simulink model "D_20210914_Modell_Inbetriebnahme_BreakOutBox_Jetson"  (R2021a)
settings: Solver=ode1  StartTime=0.0  StopTime=500  FixedStep=Ts  RelTol=1e-3
PreLoadFcn:
  | pulsePeriod = 0.05;
  | 
  | Ts = 0.001;
  | 
  | FPGA_Frequency = 75000000;
  | 
  | ts_IO691 = 5e-3;
PostLoadFcn:
  | ewolfSetUp
InitFcn:
  | pulsePeriod = 0.05;
  | 
  | Ts = 0.001;
  | 
  | FPGA_Frequency = 75000000;
  | 
  | ts_IO691 = 5e-3;
StopFcn:
  | Simulink.sdi.clearPreferences;
  | if isfile(['sdi_view_',bdroot,'.mldatx'])
  | Simulink.sdi.view;
  | pause(3);
  | Simulink.sdi.loadView(['sdi_view_',bdroot,]);
  | end
values from neighbouring files (symbols this model uses):
  max_ac = 2    [ewolfSetUp.m]
  max_steer = 0.26    [ewolfSetUp.m]
  min_ac = -3    [ewolfSetUp.m]
  min_steer = -0.26    [ewolfSetUp.m]
  PredictionHorizon = 30    [ewolfSetUp.m]
undefined symbols (not defined in the file or in its folder): canChannel, DiscIntNeverNeededParam, Ended, HS, IO291, IO397, Single
libraries: lllalib x255, canmsglib x143, simulink x33, speedgoatlib_IO191 x5, speedgoatlib_IO291 x5, speedgoatlib_IO691 x3, slrealtimeiplib x2, simulink_extras x1, speedgoatlib_fpga_dio x1, speedgoatlib_fpga_quadrature x1, speedgoatlib_fpga x1, canlib x1
(part 1 of 7)
settings Model: SimulationMode=external  ExtModeEnableFloating=off  Creator=daniel.carretero  LastModifiedBy=gao
settings SolverCC: ConcurrentTasks=on  PositivePriorityOrder=on  AutoInsertRateTranBlk=on
settings DataIOCC: ReturnWorkspaceOutputs=off
settings OptimizationCC: BlockReduction=off  OptimizeBlockIOStorage=off
settings DebuggingCC: TasksWithSamePriorityMsg=none  UnconnectedInputMsg=none  UnconnectedOutputMsg=none  UnconnectedLineMsg=none
settings HardwareCC: ProdBitPerLong=64  ProdLongLongMode=on  ProdHWDeviceType=Intel->x86-64 (Linux 64)
settings RTWCC: Description=Simulink Real-Time  SystemTargetFile=slrealtime.tlc  TemplateMakefile=slrealtime_default_tmf  RTWVerbose=off  Toolchain=Simulink Real-Time Toolchain  BuildConfiguration=Faster Runs  CodeExecutionProfiling=on  TargetLang=C++

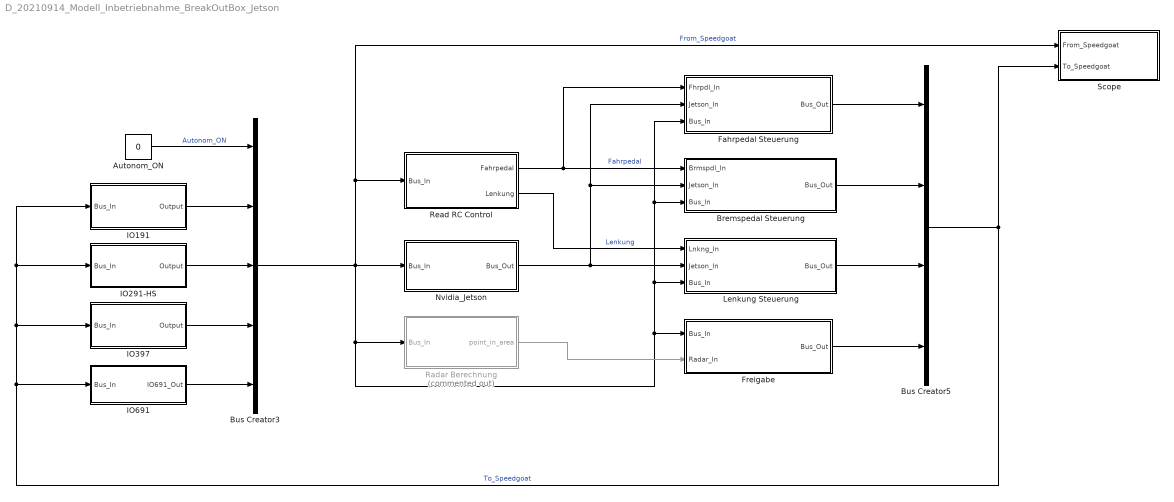
== system D_20210914_Modell_Inbetriebnahme_BreakOutBox_Jetson ==
  Autonom_ON : Constant  Value=0
  Bremspedal Steuerung : Subsystem
  Bus Creator3 : BusCreator  Inputs=5
  Bus Creator5 : BusCreator  Inputs=4
  Fahrpedal Steuerung : Subsystem
  Freigabe : Subsystem
  IO191 : Subsystem
  IO291-HS : Subsystem
  IO397 : Subsystem
  IO691 : Subsystem
  Lenkung Steuerung : Subsystem
  Nvidia_Jetson : Subsystem
  Radar Berechnung : Subsystem  Description=|  Commented=on
      | Extract radar data from CAN messages and create vector object with: 1788 fields:
      | 
      | 1. Timestamp
      | 2. cycle_count
      | 3. number of Objects
      | 4. radar timestamp_header
      | 5. CAN ID
      | +++++++++++++++++++++
      | % last point
      | 6. range
      | 7. az
      | 8. vr
      | 9. rcs
      | 10. el
      | ----------------------------------
      | % last point -1
      | 11. range
      | 12. az
      | 13. vr
      | 14. rcs
      | 15. el
      |  ...
      | 
      | empty points, all values == 0
  Read RC Control : Subsystem
  Scope : Subsystem
  wires:
  IO191/1(Output) -> Bus Creator3/2
  IO291-HS/1(Output) -> Bus Creator3/3
  IO397/1(Output) -> Bus Creator3/4
  Read RC Control/2(Lenkung) -> Lenkung Steuerung/1(Lnkng_In)  "Lenkung"
  Bus Creator3/1 -> Scope/1(From_Speedgoat), Read RC Control/1(Bus_In), Radar Berechnung/1(Bus_In), Fahrpedal Steuerung/3(Bus_In), Bremspedal Steuerung/3(Bus_In), Lenkung Steuerung/3(Bus_In), Freigabe/1(Bus_In), Nvidia_Jetson/1(Bus_In)  "From_Speedgoat"
  Read RC Control/1(Fahrpedal) -> Bremspedal Steuerung/1(Brmspdl_In), Fahrpedal Steuerung/1(Fhrpdl_In)  "Fahrpedal"
  IO691/1(IO691_Out) -> Bus Creator3/5
  Fahrpedal Steuerung/1(Bus_Out) -> Bus Creator5/1
  Lenkung Steuerung/1(Bus_Out) -> Bus Creator5/3
  Freigabe/1(Bus_Out) -> Bus Creator5/4
  Bremspedal Steuerung/1(Bus_Out) -> Bus Creator5/2
  Bus Creator5/1 -> IO191/1(Bus_In), IO291-HS/1(Bus_In), IO397/1(Bus_In), IO691/1(Bus_In), Scope/2(To_Speedgoat)  "To_Speedgoat"
  Nvidia_Jetson/1(Bus_Out) -> Fahrpedal Steuerung/2(Jetson_In), Bremspedal Steuerung/2(Jetson_In), Lenkung Steuerung/2(Jetson_In)
  Autonom_ON/1 -> Bus Creator3/1  "Autonom_ON"
  Radar Berechnung/1(point_in_area) -> Freigabe/2(Radar_In)

== system D_20210914_Modell_Inbetriebnahme_BreakOutBox_Jetson/Bremspedal Steuerung ==
  Brmspdl_In : Inport
  Jetson_In : Inport  Port=2
  Bus_In : Inport  Port=3
  1-D Lookup Table2 : Lookup_n-D  NumberOfTableDimensions=1  BreakpointsForDimension1=[min_ac max_ac]  Table=[-1 1]  InternalRulePriority=Speed  RndMeth=Simplest  InputSameDT=on
  AND3 : Logic  Inputs=3  AllPortsSameDT=off  OutDataTypeStr=boolean
  AND4 : Logic  Inputs=3  AllPortsSameDT=off  OutDataTypeStr=boolean
  Bus Creator : BusCreator  Inputs=2
  Bus Selector : BusSelector  OutputSignals=IO291_Out.IO291_Iso_DI.IO291_DI_CH1_NotAus_1,IO291_Out.IO291_Iso_DI.IO291_DI_CH2_NotAus_2,IO397_Out.IO397_DIO.IO397_DI_Ch8_Bremsaktuator_Hall_1,IO397_Out.IO397_DIO.IO397_DI_Ch9_Bremsaktuator_Hall_2,IO397_Out.IO397_QAD.IO397_QAD_Turns,Autonom_ON
  Bus Selector1 : BusSelector  OutputSignals=acceleration
  Gain : Gain  Gain=-1
  Moving Average : Subsystem
  Moving Average1 : Subsystem
  QAD Steuerung : Subsystem  Commented=on
  QAD Steuerung1 : Subsystem
  Saturation3 : Saturate  UpperLimit=0  LowerLimit=-1
  Switch : Switch  Criteria=u2 > Threshold  Threshold=0.5
  Bus_Out : Outport
  wires:
  Brmspdl_In/1 -> Switch/3
  Saturation3/1 -> Gain/1
  Bus_In/1 -> Bus Selector/1
  Bus Selector/2 -> AND4/2, AND3/2  "<IO291_DI_CH2_NotAus_2>"
  Bus Selector/1 -> AND4/1, AND3/1  "<IO291_DI_CH1_NotAus_1>"
  AND3/1 -> Bus Creator/1  "Bremsaktuator_1"
  AND4/1 -> Bus Creator/2  "Bremsaktuator_2"
  Bus Selector/5 -> QAD Steuerung/1(<QAD_Turns>)  "<IO397_QAD_Turns>"
  Gain/1 -> QAD Steuerung1/3(Brk), QAD Steuerung/2(u)
  Bus Selector/3 -> Moving Average/1(In)  "<IO397_DI_Ch8_Bremsaktuator_Hall_1>"
  Bus Selector/4 -> Moving Average1/1(In)  "<IO397_DI_Ch9_Bremsaktuator_Hall_2>"
  Moving Average/1(Hall_A) -> QAD Steuerung1/1(Hall_A)  "Hall_A"
  Moving Average1/1(Hall_B) -> QAD Steuerung1/2(Hall_B)  "Hall_B"
  QAD Steuerung1/1(Rel_1) -> AND3/3  "Rel_1"
  QAD Steuerung1/2(Rel_2) -> AND4/3  "Rel_2"
  Bus Creator/1 -> Bus_Out/1  "Brmskttr"
  Jetson_In/1 -> Bus Selector1/1
  Bus Selector1/1 -> 1-D Lookup Table2/1  "<acceleration>"
  Bus Selector/6 -> Switch/2  "<Autonom_ON>"
  Switch/1 -> Saturation3/1
  1-D Lookup Table2/1 -> Switch/1

== system D_20210914_Modell_Inbetriebnahme_BreakOutBox_Jetson/Fahrpedal Steuerung ==
  Fhrpdl_In : Inport
  Jetson_In : Inport  Port=2
  Bus_In : Inport  Port=3
  1-D Lookup Table : Lookup_n-D  NumberOfTableDimensions=1  BreakpointsForDimension1=[0:1]  Table=[0.8 5]  InternalRulePriority=Speed  RndMeth=Simplest  InputSameDT=on
  1-D Lookup Table1 : Lookup_n-D  NumberOfTableDimensions=1  BreakpointsForDimension1=[0:1]  Table=[0.4 2.5]  InternalRulePriority=Speed  RndMeth=Simplest  InputSameDT=on
  1-D Lookup Table2 : Lookup_n-D  NumberOfTableDimensions=1  BreakpointsForDimension1=[min_ac max_ac]  Table=[-1 1]  InternalRulePriority=Speed  RndMeth=Simplest  InputSameDT=on
  Bias1 : Bias
  Bias2 : Bias
  Bus Creator : BusCreator  Inputs=2
  Bus Selector : BusSelector  OutputSignals=acceleration
  Bus Selector1 : BusSelector  OutputSignals=Autonom_ON
  IC2 : InitialCondition  Value=0.8
  IC3 : InitialCondition  Value=0.4
  Saturation3 : Saturate  UpperLimit=1  LowerLimit=0
  Switch : Switch  Criteria=u2 > Threshold  Threshold=0.5
  Bus_Out : Outport
  wires:
  Bias1/1 -> Bus Creator/1  "Ausgabe_Gaspedal_FP_1_G"
  Bias2/1 -> Bus Creator/2  "Ausgabe_Gaspedal_FP_2_G"
  IC2/1 -> Bias1/1
  IC3/1 -> Bias2/1
  1-D Lookup Table/1 -> IC2/1
  Saturation3/1 -> 1-D Lookup Table1/1, 1-D Lookup Table/1
  1-D Lookup Table1/1 -> IC3/1
  Bus Creator/1 -> Bus_Out/1  "Fhrpdl"
  Jetson_In/1 -> Bus Selector/1
  Bus Selector/1 -> 1-D Lookup Table2/1  "<acceleration>"
  Bus_In/1 -> Bus Selector1/1
  Bus Selector1/1 -> Switch/2  "<Autonom_ON>"
  Fhrpdl_In/1 -> Switch/3
  Switch/1 -> Saturation3/1
  1-D Lookup Table2/1 -> Switch/1

== system D_20210914_Modell_Inbetriebnahme_BreakOutBox_Jetson/Freigabe ==
  Bus_In : Inport
  Radar_In : Inport  Port=2
  Bus Creator : BusCreator  Inputs=8
  Constant13 : Constant
  Constant8 : Constant  Value=0
  Freigabe : Subsystem
  Gain{4..9} (6 alike) : Gain
  Terminator : Terminator
  Totmann : Subsystem
  Bus_Out : Outport
  wires:
  Totmann/1(Totmann_Freigabe) -> Freigabe/2(Totmann_In)
  Bus_In/1 -> Freigabe/1(Bus_In), Totmann/1(Bus_In)
  Totmann/2(Totmann_LED) -> Gain4/1
  Gain4/1 -> Bus Creator/7  "LED_Totmann"
  Gain8/1 -> Bus Creator/3  "LG_FET_1_On"
  Gain9/1 -> Bus Creator/4  "LG_FET_2_On"
  Gain7/1 -> Bus Creator/2  "FP_FET_2_On"
  Gain5/1 -> Bus Creator/6  "Taster_Freigabe"
  Freigabe/1(Freigabe_Out) -> Gain5/1, Gain9/1, Gain8/1, Gain7/1, Gain6/1
  Constant8/1 -> Bus Creator/5  "Br_Licht_On"
  Gain6/1 -> Bus Creator/1  "FP_FET_1_On"
  Bus Creator/1 -> Bus_Out/1  "Freigabe"
  Constant13/1 -> Bus Creator/8  "USS_Reverse"
  Radar_In/1 -> Terminator/1

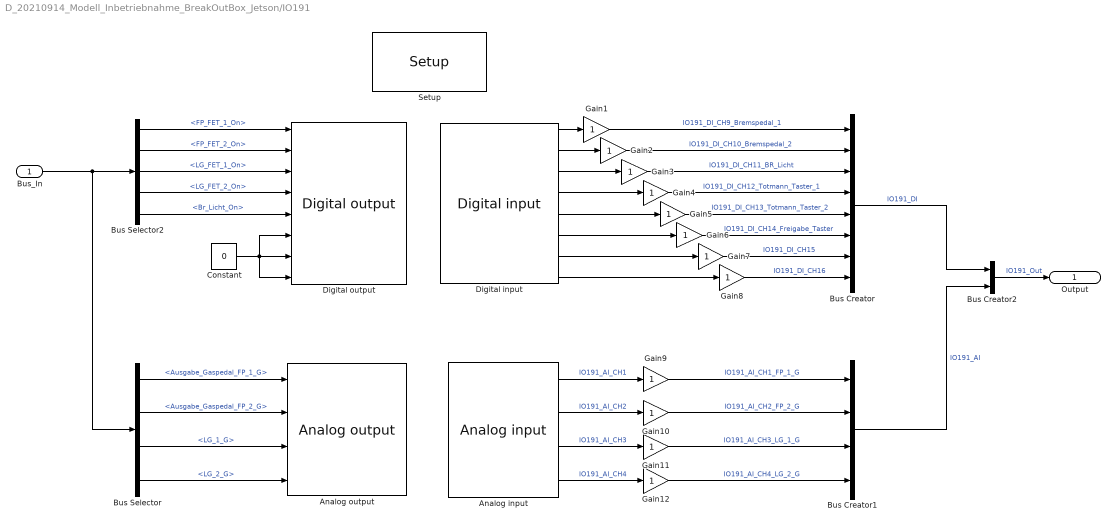
== system D_20210914_Modell_Inbetriebnahme_BreakOutBox_Jetson/IO191 ==
  Bus_In : Inport
  "Analog input " : speedgoatlib_IO191/Analog input   parModuleId=1  parSampleTime=Ts  parPciSlot=-1  parAdcChannels=[1 2 3 4]  parAdcMode=2  parAdcRanges=[4 4 4 4]  parAdcRate=100000  parAdcInitValues=[0 0]  parAdcResets=[1 1]
      settings: SourceProductName=Simulink Real-Time: Speedgoat I/O Blockset
  "Analog output " : speedgoatlib_IO191/Analog output   parModuleId=1  parSampleTime=Ts  parPciSlot=-1  parDacChannels=[1 2 3 4]  parModuleType=1  parDacRanges=[1 1 1 1]  parDacInitValues=[0 0 2.5 2.5]  parDacResets=[1 1 1 1]
      settings: SourceProductName=Simulink Real-Time: Speedgoat I/O Blockset
  Bus Creator : BusCreator  Inputs=8
  Bus Creator1 : BusCreator  Inputs=4
  Bus Creator2 : BusCreator  Inputs=2
  Bus Selector : BusSelector  OutputSignals=Fhrpdl.Ausgabe_Gaspedal_FP_1_G,Fhrpdl.Ausgabe_Gaspedal_FP_2_G,Lnkng.LG_1_G,Lnkng.LG_2_G
  Bus Selector2 : BusSelector  OutputSignals=Freigabe.FP_FET_1_On,Freigabe.FP_FET_2_On,Freigabe.LG_FET_1_On,Freigabe.LG_FET_2_On,Freigabe.Br_Licht_On
  Constant : Constant  Value=0
  "Digital input " : speedgoatlib_IO191/Digital input   parModuleId=1  parSampleTime=Ts  parPciSlot=-1  parDiChannels=[9 10 11 12 13 14 15 16]
      settings: SourceProductName=Simulink Real-Time: Speedgoat I/O Blockset
  "Digital output " : speedgoatlib_IO191/Digital output   parModuleId=1  parSampleTime=Ts  parPciSlot=-1  parDoChannels=[1 2 3 4 5 6 7 8]  parDoInitValues=[0 0 0 0 0 0 0 0]  parDoResets=[1 1 1 1 1 1 1 1]
      settings: SourceProductName=Simulink Real-Time: Speedgoat I/O Blockset
  Gain{1..12} (12 alike) : Gain
  "Setup " : speedgoatlib_IO191/Setup   parModuleId=1  parPciSlot=-1  parTriggerSignal=TTL  parAdcChannels=[1 2 3 4]  parAdcRanges=[4 4 4 4]  parAdcChannel1=on  parAdcChannel2=on  parAdcChannel3=on  parAdcChannel4=on  parAdcChannel5=off  parAdcChannel6=off  parAdcChannel7=off  parAdcChannel8=off  parAdcMode=Single-Ended  parAdcRate=100000  parAdcRange11=+-5.12 V  parAdcRange21=+-24.576 V  parAdcRange12=+-5.12 V  parAdcRange22=+-24.576 V  parAdcRange13=+-5.12 V  parAdcRange23=+-24.576 V  parAdcRange14=+-5.12 V  parAdcRange24=+-24.576 V  parAdcRange15=+-10.24 V  parAdcRange25=+-24.576 V  parAdcRange16=+-10.24 V  parAdcRange26=+-24.576 V  parAdcRange17=+-10.24 V  parAdcRange27=+-24.576 V  parAdcRange18=+-10.24 V  parAdcRange28=+-24.576 V  parDacChannels=[1 2 3 4]  parDacChannel1=on  parDacChannel2=on  parDacChannel3=on  parDacChannel4=on  parDacMode=Single-Ended  parDacRanges=[1 1 1 1]  parDacInitValues=[0 0 2.5 2.5]  parDacResets=[1 1 1 1]  parDacRange1=0 V to 5 V  parDacInitValue1=0  parDacReset1=on  parDacRange2=0 V to 5 V  parDacInitValue2=0  parDacReset2=on  parDacRange3=0 V to 5 V  parDacInitValue3=2.5  parDacReset3=on  parDacRange4=0 V to 5 V  parDacInitValue4=2.5  parDacReset4=on  parDiChannels=[9 10 11 12 13 14 15 16]  parDoChannels=[1 2 3 4 5 6 7 8]  parDioFirstControl=1  parDioSecondControl=0  parDioChannel1=Out  parExtra1=I  parExtra2=I  parExtra3=I  parDioChannel2=In  parDioChannel3=In  parDioChannel4=In  parDioChannel5=In  parDioChannel6=In  parDioChannel7=In  parDioChannel8=In  parDioChannel9=In  parDoInitValues=[0 0 0 0]  parDoResets=[1 1 1 1]  parDoInitValue1=0  parDoReset1=on  parDoInitValue2=0  parDoReset2=on  parDoInitValue3=0  parDoReset3=on  parDoInitValue4=0  parDoReset4=on  parDoInitValue5=0  parDoReset5=on  parDoInitValue6=0  parDoReset6=on  parDoInitValue7=0  parDoReset7=on  parDoInitValue8=0  parDoReset8=on  parDoInitValue9=0  parDoReset9=on  parDoInitValue10=0  parDoReset10=on  parDoInitValue11=0  parDoReset11=on  parDoInitValue12=0  parDoReset12=on  parDoInitValue13=0  parDoReset13=on  parDoInitValue14=0  parDoReset14=on  parDoInitValue15=0  parDoReset15=on  parDoInitValue16=0  parDoReset16=on
      settings: SourceProductName=Simulink Real-Time: Speedgoat I/O Blockset
  Output : Outport
  wires:
  "Digital input "/7 -> Gain7/1
  "Digital input "/1 -> Gain1/1
  "Digital input "/6 -> Gain6/1
  "Digital input "/8 -> Gain8/1
  "Digital input "/5 -> Gain5/1
  "Digital input "/4 -> Gain4/1
  "Digital input "/3 -> Gain3/1
  "Digital input "/2 -> Gain2/1
  Gain1/1 -> Bus Creator/1  "IO191_DI_CH9_Bremspedal_1"
  Gain2/1 -> Bus Creator/2  "IO191_DI_CH10_Bremspedal_2"
  Gain3/1 -> Bus Creator/3  "IO191_DI_CH11_BR_Licht"
  Gain4/1 -> Bus Creator/4  "IO191_DI_CH12_Totmann_Taster_1"
  Gain5/1 -> Bus Creator/5  "IO191_DI_CH13_Totmann_Taster_2"
  Gain6/1 -> Bus Creator/6  "IO191_DI_CH14_Freigabe_Taster"
  Gain7/1 -> Bus Creator/7  "IO191_DI_CH15"
  Gain8/1 -> Bus Creator/8  "IO191_DI_CH16"
  "Analog input "/1 -> Gain9/1  "IO191_AI_CH1"
  "Analog input "/2 -> Gain10/1  "IO191_AI_CH2"
  "Analog input "/3 -> Gain11/1  "IO191_AI_CH3"
  "Analog input "/4 -> Gain12/1  "IO191_AI_CH4"
  Bus Creator/1 -> Bus Creator2/1  "IO191_DI"
  Bus Creator1/1 -> Bus Creator2/2  "IO191_AI"
  Bus Creator2/1 -> Output/1  "IO191_Out"
  Gain9/1 -> Bus Creator1/1  "IO191_AI_CH1_FP_1_G"
  Gain10/1 -> Bus Creator1/2  "IO191_AI_CH2_FP_2_G"
  Gain11/1 -> Bus Creator1/3  "IO191_AI_CH3_LG_1_G"
  Gain12/1 -> Bus Creator1/4  "IO191_AI_CH4_LG_2_G"
  Constant/1 -> "Digital output "/6, "Digital output "/8, "Digital output "/7
  Bus_In/1 -> Bus Selector/1, Bus Selector2/1
  Bus Selector2/1 -> "Digital output "/1  "<FP_FET_1_On>"
  Bus Selector2/2 -> "Digital output "/2  "<FP_FET_2_On>"
  Bus Selector2/3 -> "Digital output "/3  "<LG_FET_1_On>"
  Bus Selector2/4 -> "Digital output "/4  "<LG_FET_2_On>"
  Bus Selector2/5 -> "Digital output "/5  "<Br_Licht_On>"
  Bus Selector/1 -> "Analog output "/1  "<Ausgabe_Gaspedal_FP_1_G>"
  Bus Selector/2 -> "Analog output "/2  "<Ausgabe_Gaspedal_FP_2_G>"
  Bus Selector/3 -> "Analog output "/3  "<LG_1_G>"
  Bus Selector/4 -> "Analog output "/4  "<LG_2_G>"

== system D_20210914_Modell_Inbetriebnahme_BreakOutBox_Jetson/IO291-HS ==
  Bus_In : Inport
  Alive : Constant  Value=0
  Bus Creator : BusCreator  Inputs=1
  Bus Creator1 : BusCreator  Inputs=2
  Bus Creator2 : BusCreator  Inputs=2
  Bus Selector1 : BusSelector  OutputSignals=Brmskttr.Bremsaktuator_1,Brmskttr.Bremsaktuator_2,Freigabe.USS_Reverse,Freigabe.LED_Totmann,Freigabe.Taster_Freigabe
  Data Type Conversion : DataTypeConversion
  Data Type Conversion1 : DataTypeConversion
  "FET digital output " : speedgoatlib_IO291/FET digital output   parModuleId=1  parSampleTime=Ts  parPciSlot=-1  parFetDoChannels=[1 2 4 5 6]  parFetDoInitValues=[0 0 0 0 0]  parFetDoReset=[1 1 1 1 1]  parModuleType=IO291-HS  parInternalModuleId=1
      settings: SourceProductName=Simulink Real-Time: Speedgoat Library
  Gain : Gain
  Gain1 : Gain
  "Isolated digital input " : speedgoatlib_IO291/Isolated digital input   parModuleId=1  parSampleTime=Ts  parPciSlot=-1  parIsolDiChannels=[1 2]  parModuleType=IO291-HS  parInternalModuleId=1
      settings: SourceProductName=Simulink Real-Time: Speedgoat Library
  "LVTTL digital input " : speedgoatlib_IO291/LVTTL digital input   parModuleId=1  parSampleTime=Ts  parPciSlot=-1  parTtlDiChannels=[]  parModuleType=IO291-HS  parInternalModuleId=1
      settings: SourceProductName=Simulink Real-Time: Speedgoat Library
  "LVTTL digital output " : speedgoatlib_IO291/LVTTL digital output   parModuleId=1  parSampleTime=Ts  parPciSlot=-1  parTtlDoChannels=[]  parTtlDoInitValues=zeros(1,0)  parTtlDoReset=zeros(1,0)  parModuleType=IO291-HS  parInternalModuleId=1
      settings: SourceProductName=Simulink Real-Time: Speedgoat Library
  "Setup " : speedgoatlib_IO291/Setup   parInternalModuleId=1  parPciSlot=-1  parModuleId=1  parModuleType=IO291-HS  parTtlDoChannels=[]  parTtlDoInitValues=0  parTtlDoReset=1  parTtlDiChannels=[]  parIsolDiChannels=[1:2]  parFetDoChannels=[1 2 4:6]  parFetDoInitValues=0  parFetDoReset=1
      settings: SourceProductName=Simulink Real-Time: Speedgoat Library
  Output : Outport
  wires:
  "Isolated digital input "/1 -> Gain/1
  "Isolated digital input "/2 -> Gain1/1
  Bus Creator/1 -> Bus Creator2/1  "IO291_LVTTL_DI"
  Bus Creator1/1 -> Bus Creator2/2  "IO291_Iso_DI"
  Bus Creator2/1 -> Output/1  "IO291_Out"
  Alive/1 -> Bus Creator/1  "Alive"
  Data Type Conversion/1 -> "FET digital output "/1
  Data Type Conversion1/1 -> "FET digital output "/2
  Gain/1 -> Bus Creator1/1  "IO291_DI_CH1_NotAus_1"
  Gain1/1 -> Bus Creator1/2  "IO291_DI_CH2_NotAus_2"
  Bus_In/1 -> Bus Selector1/1
  Bus Selector1/1 -> Data Type Conversion/1  "<Bremsaktuator_1>"
  Bus Selector1/2 -> Data Type Conversion1/1  "<Bremsaktuator_2>"
  Bus Selector1/3 -> "FET digital output "/3  "<USS_Reverse>"
  Bus Selector1/4 -> "FET digital output "/4  "<LED_Totmann>"
  Bus Selector1/5 -> "FET digital output "/5  "<Taster_Freigabe>"

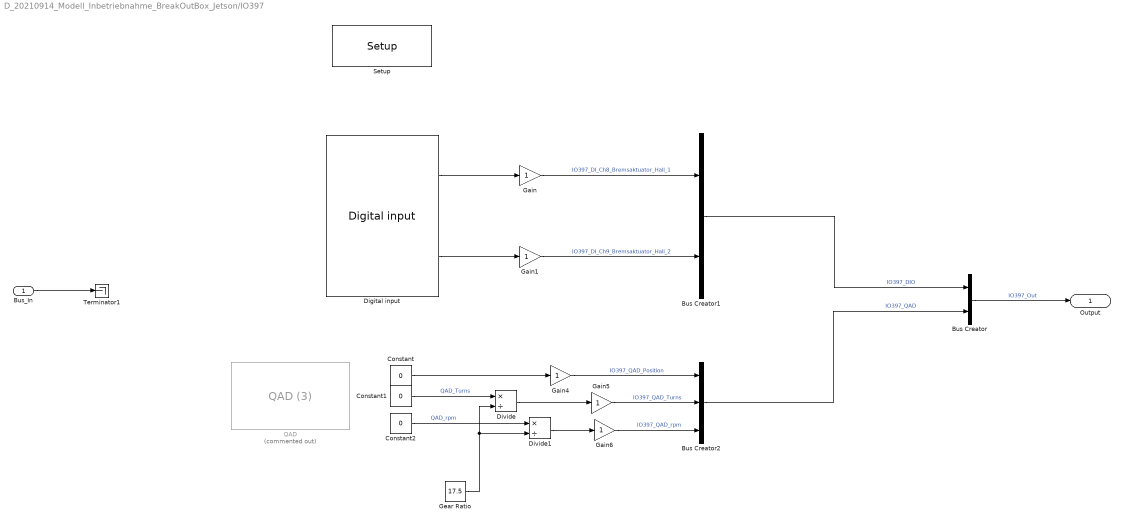
== system D_20210914_Modell_Inbetriebnahme_BreakOutBox_Jetson/IO397 ==
  Bus_In : Inport
  Bus Creator : BusCreator  Inputs=2
  Bus Creator1 : BusCreator  Inputs=2
  Bus Creator2 : BusCreator  Inputs=3
  Constant : Constant  Value=0
  Constant1 : Constant  Value=0
  Constant2 : Constant  Value=0
  Digital input : speedgoatlib_fpga_dio/Digital input  id=1  chan=[8,9]  ts=Ts  pciSlot=-1  board=IO397-50k  vectorizeOutput=off
      settings: SourceProductName=Simulink Real-Time: Speedgoat I/O Driver Library
  Divide : Product  Inputs=*/
  Divide1 : Product  Inputs=*/
  Gain{,1,4..6} (5 alike) : Gain
  Gear Ratio : Constant  Value=17.5
  QAD : speedgoatlib_fpga_quadrature/QAD (3)  Commented=on  id=1  board=IO397-50k  chan=1  resetOnStart=on  ts=Ts  pciSlot=-1  operatingMode=Quadrature decoder  indexControlMode=Ignore index  resolution=4x  stepsPerRevolution=12  latchMode=Disabled  interpolatePosition=off  invertAB=off  showClearPositionInput=off  showClearIndexFoundInput=off  showPositionOutput=on  showTurnOutput=on  showSpeedOutput=on  showDirectionOutput=off  showIndexFoundOutput=off
      settings: SourceProductName=Simulink Real-Time: Speedgoat I/O Driver Library
  Setup : speedgoatlib_fpga/Setup/Setup  board=IO397-50k  id=1  device_id=1  frontIO=None  rearIO=None  bitstreamFile=speedgoat_IO397_50k_Comms.mat  rev=2.000000  timestamp_string=15/09/21 23:42:36  fpgaFreq=75 MHz  fpgaTick=13.33 ns  ProgSpiFlash=off  ProgBPIFlash=off  pciSlot=-1  PullRPort0=pull-up 3.3V  VioPort0=3.3V  PullRPort1=pull-up 3.3V  VioPort1=3.3V  PullRPort2=pull-up 3.3V  VioPort2=3.3V  PullRPort3=pull-up 3.3V  VioPort3=3.3V  PullRPort4=pull-up 3.3V  VioPort4=3.3V  PullRPort5=pull-up 3.3V  VioPort5=3.3V  PullRPort6=pull-up 3.3V  VioPort6=3.3V  PullRPort15=pull-down  PullRPort31=pull-up 3.3V  PullRPort47=pull-up 3.3V  PullRPort63=pull-up 3.3V
      settings: SourceProductName=Simulink Real-Time: Speedgoat Library
  Terminator1 : Terminator
  Output : Outport
  wires:
  Bus Creator/1 -> Output/1  "IO397_Out"
  Constant/1 -> Gain4/1
  Bus Creator1/1 -> Bus Creator/1  "IO397_DIO"
  Bus Creator2/1 -> Bus Creator/2  "IO397_QAD"
  Divide/1 -> Gain5/1
  Divide1/1 -> Gain6/1
  Gear Ratio/1 -> Divide1/2, Divide/2
  Constant1/1 -> Divide/1  "QAD_Turns"
  Constant2/1 -> Divide1/1  "QAD_rpm"
  Digital input/2 -> Gain1/1
  Digital input/1 -> Gain/1
  Gain/1 -> Bus Creator1/1  "IO397_DI_Ch8_Bremsaktuator_Hall_1"
  Gain1/1 -> Bus Creator1/2  "IO397_DI_Ch9_Bremsaktuator_Hall_2"
  Gain4/1 -> Bus Creator2/1  "IO397_QAD_Position"
  Gain5/1 -> Bus Creator2/2  "IO397_QAD_Turns"
  Gain6/1 -> Bus Creator2/3  "IO397_QAD_rpm"
  Bus_In/1 -> Terminator1/1

== system D_20210914_Modell_Inbetriebnahme_BreakOutBox_Jetson/IO691 ==
  note: PORT 1 - RX
  note: PORT 2 - RX
  Bus_In : Inport
  Bus Creator : BusCreator  Inputs=2
  CAN Read Loop - Port 1 : Subsystem  TreatAsAtomicUnit=on
  CAN Read Loop - Port 3 : Subsystem  TreatAsAtomicUnit=on
  "CAN Setup " : speedgoatlib_IO691/CAN Setup   moduletype=IO691  id=1  pciSlot=-1  chn1=CAN (HS)  chn2=CAN (HS)  chn3=Disabled  chn4=Disabled  initStruct=[]  termStruct=[]  ArbitrationbdrChn1=500 kBaud  ArbitrationManbdrChn1=[2,16,63,16]  FdbdrChn1=5.0 MBaud  FdManbdrChn1=[2,2,5,2]  ArbitrationbdrChn2=500 kBaud  ArbitrationManbdrChn2=[2,16,63,16]  FdbdrChn2=5.0 MBaud  FdManbdrChn2=[2,2,5,2]  ArbitrationbdrChn3=1.0 MBaud  ArbitrationManbdrChn3=[2,8,31,8]  FdbdrChn3=5.0 MBaud  FdManbdrChn3=[2,2,5,2]  ArbitrationbdrChn4=1.0 MBaud  ArbitrationManbdrChn4=[2,8,31,8]  FdbdrChn4=5.0 MBaud  FdManbdrChn4=[2,2,5,2]  moduleInitValues=[691 1 -1 -1]
      settings: SourceProductName=Simulink Real-Time: Speedgoat Library
  RX Sample Time : Constant  SampleTime=ts_IO691
  Terminator1 : Terminator
  IO691_Out : Outport
  wires:
  RX Sample Time/1 -> CAN Read Loop - Port 3/1(SampleTime), CAN Read Loop - Port 1/1(SampleTime)
  Bus Creator/1 -> IO691_Out/1  "IO691_Out"
  CAN Read Loop - Port 1/1(CAN_Out) -> Bus Creator/2  "IO691_CAN_eWolf"
  CAN Read Loop - Port 3/1(CAN_Out) -> Bus Creator/1  "IO691_CAN_Sensoren"
  Bus_In/1 -> Terminator1/1

== system D_20210914_Modell_Inbetriebnahme_BreakOutBox_Jetson/Lenkung Steuerung ==
  Lnkng_In : Inport
  Jetson_In : Inport  Port=2
  Bus_In : Inport  Port=3
  1-D Lookup Table : Lookup_n-D  NumberOfTableDimensions=1  BreakpointsForDimension1=[0:1]  Table=[1.6 3.4]  InternalRulePriority=Speed  RndMeth=Simplest  InputSameDT=on
  1-D Lookup Table1 : Lookup_n-D  NumberOfTableDimensions=1  BreakpointsForDimension1=[0:1]  Table=[3.4 1.6]  InternalRulePriority=Speed  RndMeth=Simplest  InputSameDT=on
  1-D Lookup Table2 : Lookup_n-D  NumberOfTableDimensions=1  BreakpointsForDimension1=[min_steer max_steer]  Table=[0 1]  InternalRulePriority=Speed  RndMeth=Simplest  InputSameDT=on
  Bias : Bias  Bias=0.25
  Bias1 : Bias  Bias=0.25
  Bus Creator : BusCreator  Inputs=2
  Bus Selector : BusSelector  OutputSignals=steering_angle
  Bus Selector1 : BusSelector  OutputSignals=Autonom_ON
  IC2 : InitialCondition  Value=2.5
  IC3 : InitialCondition  Value=2.5
  Saturation2 : Saturate  UpperLimit=1  LowerLimit=0
  Switch : Switch  Criteria=u2 > Threshold  Threshold=0.5
  Bus_Out : Outport
  wires:
  1-D Lookup Table/1 -> IC2/1
  IC2/1 -> Bias/1
  Bias1/1 -> Bus Creator/2  "LG_2_G"
  Bias/1 -> Bus Creator/1  "LG_1_G"
  IC3/1 -> Bias1/1
  1-D Lookup Table1/1 -> IC3/1
  Saturation2/1 -> 1-D Lookup Table1/1, 1-D Lookup Table/1
  Lnkng_In/1 -> Switch/3
  Bus Creator/1 -> Bus_Out/1  "Lnkng"
  Jetson_In/1 -> Bus Selector/1
  Bus Selector/1 -> 1-D Lookup Table2/1  "<steering_angle>"
  Bus_In/1 -> Bus Selector1/1
  Bus Selector1/1 -> Switch/2  "<Autonom_ON>"
  Switch/1 -> Saturation2/1
  1-D Lookup Table2/1 -> Switch/1

== system D_20210914_Modell_Inbetriebnahme_BreakOutBox_Jetson/Nvidia_Jetson ==
  Bus_In : Inport
  Bus Creator : BusCreator  Inputs=2
  Bus Selector1 : BusSelector  OutputSignals=IO691_Out.IO691_CAN_Sensoren.Radar.radar data (length 1788),IO691_Out.IO691_CAN_Sensoren.Lenkwinkel,IO691_Out.IO691_CAN_eWolf.CarSpeed
  Byte Packing : slrealtimeutilitieslib/Byte Packing  MaskPackedDataType=uint8  MaskUnpackedDataTypes={['double'],['double']}  MaskAlignment=1
  Data Type Conversion : DataTypeConversion
  From Jetson : slrealtimeiplib/UDP Receive  useHostTargetConn=off  ipAddress=10.41.0.10  localPort=5500  rcvWidth=48  rcvFmAny=on  fmAddress=10.10.10.10  sampleTime=-1
      settings: SourceProductBaseCode=XP
  LaneFollowingAndControl : Subsystem
  MATLAB Function : MATLAB Function  TreatAsAtomicUnit=on
  PackLaneBus : MATLABSystem  System=packLaneMarkerBus  Camera=camera  SimulateUsing=Code generation
      mask Type: packLaneMarkerBus
      mask Display:
      | disp('packLaneMarkerBus');
      | port_label('input',1,'msgs');
      | port_label('output',1,'lanes');
  Rate Transition1 : RateTransition
  Rate Transition2 : RateTransition
  Set Velocity : Constant  Value=5  OutDataTypeStr=single
  Terminator : Terminator
  Terminator1 : Terminator
  Terminator3 : Terminator
  To Jetson : slrealtimeiplib/UDP Send  useHostTargetConn=off  ipAddress=10.41.0.10  localPort=5500  toAddress=10.41.0.12  toPort=8080  sampleTime=-1
      settings: SourceProductBaseCode=XP
  Width : Width
  Bus_Out : Outport
  wires:
  Bus Selector1/3 -> Rate Transition1/1  "<CarSpeed>"
  LaneFollowingAndControl/2(acceleration) -> Bus Creator/2, Byte Packing/2  "acceleration"
  Rate Transition2/1 -> Terminator/1  "Lenkwinkel"
  Rate Transition1/1 -> LaneFollowingAndControl/2(Longitudinal_Velocity)  "Longitudinal_Velocity"
  Bus_In/1 -> Bus Selector1/1
  Byte Packing/1 -> Width/1, To Jetson/1
  LaneFollowingAndControl/1(steering_angle) -> Bus Creator/1, Byte Packing/1  "steering_angle"
  Width/1 -> To Jetson/2
  From Jetson/2 -> Terminator3/1
  Bus Selector1/2 -> Rate Transition2/1  "<Lenkwinkel>"
  From Jetson/1 -> PackLaneBus/1
  PackLaneBus/1 -> LaneFollowingAndControl/3(Lane Detections)
  Set Velocity/1 -> LaneFollowingAndControl/1(Set velocity)
  Bus Creator/1 -> Bus_Out/1  "Nvidia_Jetson"
  Bus Selector1/1 -> Data Type Conversion/1  "<radar data (length 1788)>"
  Data Type Conversion/1 -> Terminator1/1  "Radar_Data"

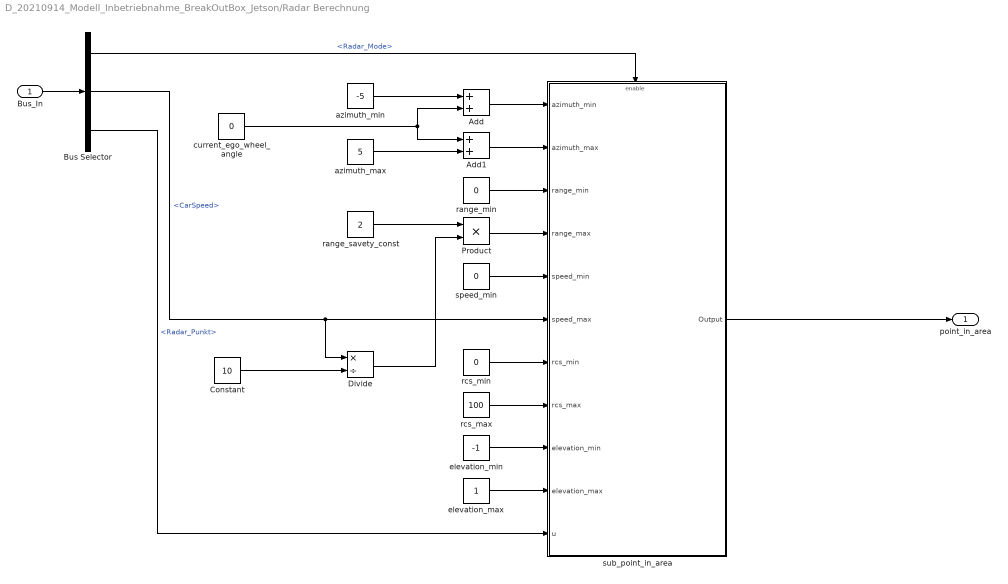
== system D_20210914_Modell_Inbetriebnahme_BreakOutBox_Jetson/Radar Berechnung ==
  Bus_In : Inport
  Add : Sum
  Add1 : Sum
  Bus Selector : BusSelector  OutputSignals=IO691_Out.IO691_CAN_Sensoren.Radar.Radar_Mode,IO691_Out.IO691_CAN_eWolf.CarSpeed,IO691_Out.IO691_CAN_Sensoren.Radar.Radar_Punkt
  Constant : Constant  Value=10
  Divide : Product  Inputs=*/
  Product : Product
  azimuth_max : Constant  Value=5
  azimuth_min : Constant  Value=-5
  current_ego_wheel_angle : Constant  Value=0
  elevation_max : Constant
  elevation_min : Constant  Value=-1
  range_min : Constant  Value=0
  range_savety_const : Constant  Value=2
  rcs_max : Constant  Value=100
  rcs_min : Constant  Value=0
  speed_min : Constant  Value=0
  sub_point_in_area : Subsystem  TreatAsAtomicUnit=on
  point_in_area : Outport
  wires:
  sub_point_in_area/1(Output) -> point_in_area/1
  rcs_max/1 -> sub_point_in_area/8(rcs_max)
  rcs_min/1 -> sub_point_in_area/7(rcs_min)
  elevation_max/1 -> sub_point_in_area/10(elevation_max)
  elevation_min/1 -> sub_point_in_area/9(elevation_min)
  Bus Selector/2 -> Divide/1, sub_point_in_area/6(speed_max)  "<CarSpeed>"
  speed_min/1 -> sub_point_in_area/5(speed_min)
  range_min/1 -> sub_point_in_area/3(range_min)
  Add/1 -> sub_point_in_area/1(azimuth_min)
  Add1/1 -> sub_point_in_area/2(azimuth_max)
  azimuth_max/1 -> Add1/2
  azimuth_min/1 -> Add/1
  current_ego_wheel_angle/1 -> Add1/1, Add/2
  Constant/1 -> Divide/2
  Divide/1 -> Product/2
  Product/1 -> sub_point_in_area/4(range_max)
  range_savety_const/1 -> Product/1
  Bus_In/1 -> Bus Selector/1
  Bus Selector/1 -> sub_point_in_area/Enable  "<Radar_Mode>"
  Bus Selector/3 -> sub_point_in_area/11(u)  "<Radar_Punkt>"

== system D_20210914_Modell_Inbetriebnahme_BreakOutBox_Jetson/Read RC Control ==
  Bus_In : Inport
  1-D Lookup Table : Lookup_n-D  NumberOfTableDimensions=1  BreakpointsForDimension1=[0 50 100]  Table=[-1 0 1]  InternalRulePriority=Speed  RndMeth=Simplest  InputSameDT=on
  Bus Selector : BusSelector  OutputSignals=IO691_Out.IO691_CAN_Sensoren.RC_Fahrpedal,IO691_Out.IO691_CAN_Sensoren.RC_Lenkung
  Compare To Constant : simulink/Logic and Bit Operations/Compare To Constant  relop===  const=255  OutDataTypeStr=boolean
  Compare To Constant1 : simulink/Logic and Bit Operations/Compare To Constant  relop===  const=255  OutDataTypeStr=boolean
  Constant : Constant  Value=50
  Constant1 : Constant  Value=50
  Constant2 : Constant  Value=100
  Divide : Product  Inputs=*/
  IC : InitialCondition  Value=0
  IC1 : InitialCondition  Value=0.5
  Saturation : Saturate  UpperLimit=100  LowerLimit=0
  Saturation1 : Saturate  UpperLimit=100  LowerLimit=0
  Switch : Switch  Criteria=u2 > Threshold  Threshold=0.5
  Switch1 : Switch  Criteria=u2 > Threshold  Threshold=0.5
  Fahrpedal : Outport
  Lenkung : Outport  Port=2
  wires:
  Bus Selector/2 -> Compare To Constant1/1, Switch1/3  "<RC_Lenkung>"
  Bus_In/1 -> Bus Selector/1
  Bus Selector/1 -> Compare To Constant/1, Switch/3  "<RC_Fahrpedal>"
  IC/1 -> Fahrpedal/1
  IC1/1 -> Lenkung/1
  Compare To Constant/1 -> Switch/2
  Constant/1 -> Switch/1
  Compare To Constant1/1 -> Switch1/2
  Constant1/1 -> Switch1/1
  Switch/1 -> Saturation/1
  Switch1/1 -> Saturation1/1
  Saturation/1 -> 1-D Lookup Table/1
  Saturation1/1 -> Divide/1
  Divide/1 -> IC1/1
  1-D Lookup Table/1 -> IC/1
  Constant2/1 -> Divide/2

== system D_20210914_Modell_Inbetriebnahme_BreakOutBox_Jetson/Scope ==
  From_Speedgoat : Inport
  To_Speedgoat : Inport  Port=2
  Bus Selector : BusSelector  OutputSignals=IO191_Out.IO191_AI.IO191_AI_CH1_FP_1_G,IO191_Out.IO191_AI.IO191_AI_CH2_FP_2_G,IO191_Out.IO191_AI.IO191_AI_CH3_LG_1_G,IO191_Out.IO191_AI.IO191_AI_CH4_LG_2_G
  Bus Selector1 : BusSelector  OutputSignals=IO691_Out.IO691_CAN_Sensoren.USS,IO691_Out.IO691_CAN_Sensoren.RC_Lenkung,IO691_Out.IO691_CAN_Sensoren.RC_Fahrpedal
  Scope : Scope  NumInputPorts=3
  Scope2 : Scope  NumInputPorts=4
  Terminator : Terminator
  wires:
  Bus Selector/2 -> Scope2/2  "<IO191_AI_CH2_FP_2_G>"
  Bus Selector/1 -> Scope2/1  "<IO191_AI_CH1_FP_1_G>"
  Bus Selector/4 -> Scope2/4  "<IO191_AI_CH4_LG_2_G>"
  From_Speedgoat/1 -> Bus Selector1/1, Bus Selector/1
  Bus Selector/3 -> Scope2/3  "<IO191_AI_CH3_LG_1_G>"
  To_Speedgoat/1 -> Terminator/1
  Bus Selector1/1 -> Scope/1  "<USS>"
  Bus Selector1/2 -> Scope/2  "<RC_Lenkung>"
  Bus Selector1/3 -> Scope/3  "<RC_Fahrpedal>"

== system D_20210914_Modell_Inbetriebnahme_BreakOutBox_Jetson/Bremspedal Steuerung/Moving Average ==
  In : Inport
  Divide : Product  Inputs=*/
  Round : Rounding  Operator=round
  Sum of Elements : Sum  Inputs=+
  Tapped Delay : simulink/Discrete/Tapped Delay  vinit=0.0  samptime=-1  NumDelays=4  DelayOrder=Oldest  includeCurrent=off
  Vector Concatenate : Concatenate
  Width : Width
  Hall_A : Outport
  wires:
  In/1 -> Vector Concatenate/1, Tapped Delay/1
  Sum of Elements/1 -> Divide/1
  Width/1 -> Divide/2
  Vector Concatenate/1 -> Sum of Elements/1, Width/1
  Divide/1 -> Round/1
  Round/1 -> Hall_A/1
  Tapped Delay/1 -> Vector Concatenate/2

== system D_20210914_Modell_Inbetriebnahme_BreakOutBox_Jetson/Bremspedal Steuerung/Moving Average1 ==
  In : Inport
  Divide : Product  Inputs=*/
  Round : Rounding  Operator=round
  Sum of Elements : Sum  Inputs=+
  Tapped Delay : simulink/Discrete/Tapped Delay  vinit=0.0  samptime=-1  NumDelays=4  DelayOrder=Oldest  includeCurrent=off
  Vector Concatenate : Concatenate
  Width : Width
  Hall_B : Outport
  wires:
  In/1 -> Vector Concatenate/1, Tapped Delay/1
  Sum of Elements/1 -> Divide/1
  Width/1 -> Divide/2
  Vector Concatenate/1 -> Sum of Elements/1, Width/1
  Divide/1 -> Round/1
  Round/1 -> Hall_B/1
  Tapped Delay/1 -> Vector Concatenate/2

== system D_20210914_Modell_Inbetriebnahme_BreakOutBox_Jetson/Bremspedal Steuerung/QAD Steuerung ==
  <QAD_Turns> : Inport
  u : Inport  Port=2
  AND : Logic  Inputs=3  AllPortsSameDT=off  OutDataTypeStr=boolean
  AND1 : Logic  AllPortsSameDT=off  OutDataTypeStr=boolean
  AND2 : Logic  AllPortsSameDT=off  OutDataTypeStr=boolean
  Compare To Constant : simulink/Logic and Bit Operations/Compare To Constant  relop=>  const=0.4  OutDataTypeStr=boolean
  Compare To Constant1 : simulink/Logic and Bit Operations/Compare To Constant  relop=<  const=0.1  OutDataTypeStr=boolean
  Compare To Constant2 : simulink/Logic and Bit Operations/Compare To Constant  relop=<  const=0  OutDataTypeStr=boolean
  Compare To Constant3 : simulink/Logic and Bit Operations/Compare To Constant  relop=>=  const=-0.2  OutDataTypeStr=boolean
  Compare To Constant4 : simulink/Logic and Bit Operations/Compare To Constant  relop=<  const=0.9  OutDataTypeStr=boolean
  Compare To Constant5 : simulink/Logic and Bit Operations/Compare To Constant  relop=>  const=0.9  OutDataTypeStr=boolean
  Compare To Constant6 : simulink/Logic and Bit Operations/Compare To Constant  relop=>=  const=-0.4  OutDataTypeStr=boolean
  IC2 : InitialCondition  Value=0
  IC3 : InitialCondition  Value=0
  OR : Logic  Operator=OR  AllPortsSameDT=off  OutDataTypeStr=boolean
  Out1 : Outport
  Out2 : Outport  Port=2
  wires:
  <QAD_Turns>/1 -> Compare To Constant3/1, Compare To Constant2/1, Compare To Constant6/1
  OR/1 -> IC2/1
  AND1/1 -> IC3/1
  IC3/1 -> Out2/1
  u/1 -> Compare To Constant5/1, Compare To Constant4/1, Compare To Constant/1, Compare To Constant1/1
  IC2/1 -> Out1/1
  Compare To Constant/1 -> AND/2
  Compare To Constant6/1 -> AND2/2
  Compare To Constant5/1 -> AND2/1
  AND/1 -> OR/1
  AND2/1 -> OR/2
  Compare To Constant3/1 -> AND/1
  Compare To Constant4/1 -> AND/3
  Compare To Constant1/1 -> AND1/2
  Compare To Constant2/1 -> AND1/1

== system D_20210914_Modell_Inbetriebnahme_BreakOutBox_Jetson/Bremspedal Steuerung/QAD Steuerung1 ==
  Hall_A : Inport
  Hall_B : Inport  Port=2
  Brk : Inport  Port=3
  1-D Lookup Table : Lookup_n-D  NumberOfTableDimensions=1  BreakpointsForDimension1=[0, 0.25, 0.5, 0.75, 1]  Table=[0, 20, 40, 60, 80]  InterpMethod=Nearest  InternalRulePriority=Speed  RndMeth=Simplest  InputSameDT=on
  AND7 : Logic  AllPortsSameDT=off  OutDataTypeStr=boolean
  AND8 : Logic  AllPortsSameDT=off  OutDataTypeStr=boolean
  Add : Sum  Inputs=-+
  Anti-Relaisprellen : Subsystem
  Compare To Constant6 : simulink/Logic and Bit Operations/Compare To Constant  relop=>  const=0.1  OutDataTypeStr=boolean
  Compare To Constant7 : simulink/Logic and Bit Operations/Compare To Constant  relop=<=  const=0  OutDataTypeStr=boolean
  Compare To Constant8 : simulink/Logic and Bit Operations/Compare To Constant  relop===  const=0  OutDataTypeStr=boolean
  Compare To Constant9 : simulink/Logic and Bit Operations/Compare To Constant  relop=>  const=0  OutDataTypeStr=boolean
  Counter : Subsystem
  QAD1 : Subsystem
  Rel_1 : Outport
  Rel_2 : Outport  Port=2
  wires:
  Hall_A/1 -> QAD1/1(Hall_A)  "Hall_A"
  Hall_B/1 -> QAD1/2(Hall_B)  "Hall_B"
  QAD1/1(Count_direction) -> Counter/1(count_dir)
  Compare To Constant6/1 -> AND7/1
  Compare To Constant7/1 -> AND7/2
  Compare To Constant8/1 -> AND8/1
  Compare To Constant9/1 -> AND8/2
  Brk/1 -> 1-D Lookup Table/1, Compare To Constant8/1, Compare To Constant6/1
  Counter/1(Value) -> Compare To Constant9/1, Add/2
  1-D Lookup Table/1 -> Add/1
  Add/1 -> Compare To Constant7/1
  QAD1/2(Count_enable) -> Counter/2(count_enable)
  AND7/1 -> Anti-Relaisprellen/1(In)
  Anti-Relaisprellen/1(Out) -> Rel_1/1
  AND8/1 -> Rel_2/1

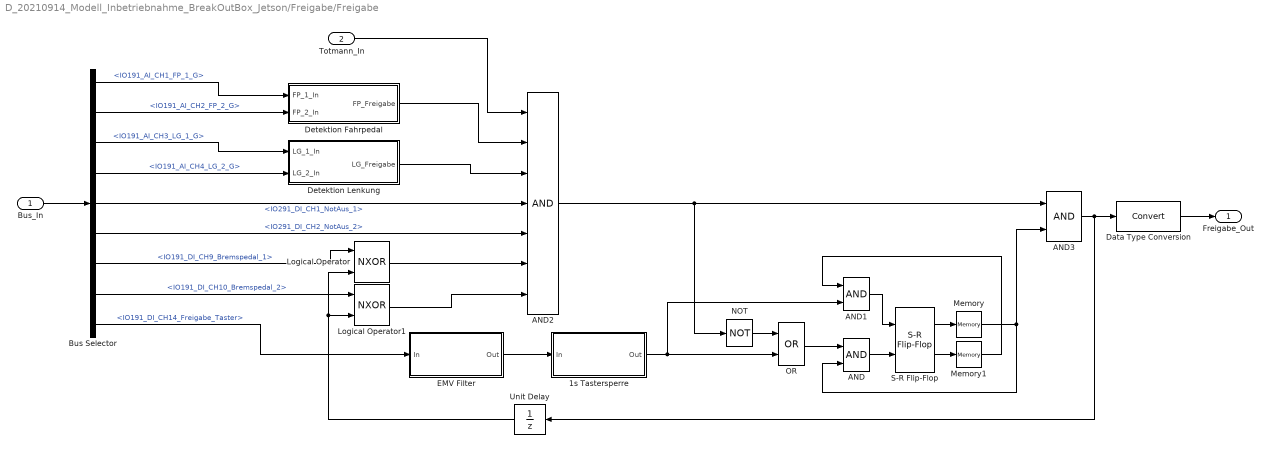
== system D_20210914_Modell_Inbetriebnahme_BreakOutBox_Jetson/Freigabe/Freigabe ==
  Bus_In : Inport
  Totmann_In : Inport  Port=2
  1s Tastersperre : Subsystem
  AND : Logic  AllPortsSameDT=off  OutDataTypeStr=boolean
  AND1 : Logic  AllPortsSameDT=off  OutDataTypeStr=boolean
  AND2 : Logic  Inputs=7  AllPortsSameDT=off  OutDataTypeStr=boolean
  AND3 : Logic  AllPortsSameDT=off  OutDataTypeStr=boolean
  Bus Selector : BusSelector  OutputSignals=IO191_Out.IO191_AI.IO191_AI_CH1_FP_1_G,IO191_Out.IO191_AI.IO191_AI_CH2_FP_2_G,IO191_Out.IO191_AI.IO191_AI_CH3_LG_1_G,IO191_Out.IO191_AI.IO191_AI_CH4_LG_2_G,IO291_Out.IO291_Iso_DI.IO291_DI_CH1_NotAus_1,IO291_Out.IO291_Iso_DI.IO291_DI_CH2_NotAus_2,IO191_Out.IO191_DI.IO191_DI_CH9_Bremspedal_1,IO191_Out.IO191_DI.IO191_DI_CH10_Bremspedal_2,IO191_Out.IO191_DI.IO191_DI_CH14_Freigabe_Taster
  Data Type Conversion : DataTypeConversion
  Detektion Fahrpedal : Subsystem
  Detektion Lenkung : Subsystem
  EMV Filter : Subsystem
  Logical Operator : Logic  Operator=NXOR  AllPortsSameDT=off  OutDataTypeStr=boolean
  Logical Operator1 : Logic  Operator=NXOR  AllPortsSameDT=off  OutDataTypeStr=boolean
  Memory : Memory  InheritSampleTime=on  LinearizeAsDelay=on
  Memory1 : Memory  InheritSampleTime=on  LinearizeAsDelay=on
  NOT : Logic  Operator=NOT  AllPortsSameDT=off  OutDataTypeStr=boolean
  OR : Logic  Operator=OR  AllPortsSameDT=off  OutDataTypeStr=boolean
  S-R Flip-Flop : simulink_extras/Flip Flops/S-R Flip-Flop  initial_condition=0
  Unit Delay : UnitDelay  SampleTime=-1  HasFrameUpgradeWarning=on
  Freigabe_Out : Outport
  wires:
  Bus_In/1 -> Bus Selector/1
  Bus Selector/9 -> EMV Filter/1(In)  "<IO191_DI_CH14_Freigabe_Taster>"
  S-R Flip-Flop/1 -> Memory/1
  AND/1 -> S-R Flip-Flop/2
  S-R Flip-Flop/2 -> Memory1/1
  AND1/1 -> S-R Flip-Flop/1
  Memory/1 -> AND3/2, AND/2
  Data Type Conversion/1 -> Freigabe_Out/1
  Memory1/1 -> AND1/1
  1s Tastersperre/1(Out) -> AND1/2, OR/2
  Totmann_In/1 -> AND2/1
  Bus Selector/1 -> Detektion Fahrpedal/1(FP_1_In)  "<IO191_AI_CH1_FP_1_G>"
  Bus Selector/2 -> Detektion Fahrpedal/2(FP_2_In)  "<IO191_AI_CH2_FP_2_G>"
  Bus Selector/3 -> Detektion Lenkung/1(LG_1_In)  "<IO191_AI_CH3_LG_1_G>"
  Bus Selector/4 -> Detektion Lenkung/2(LG_2_In)  "<IO191_AI_CH4_LG_2_G>"
  Detektion Fahrpedal/1(FP_Freigabe) -> AND2/2
  Detektion Lenkung/1(LG_Freigabe) -> AND2/3
  Bus Selector/5 -> AND2/4  "<IO291_DI_CH1_NotAus_1>"
  Bus Selector/6 -> AND2/5  "<IO291_DI_CH2_NotAus_2>"
  AND2/1 -> NOT/1, AND3/1
  AND3/1 -> Unit Delay/1, Data Type Conversion/1
  OR/1 -> AND/1
  NOT/1 -> OR/1
  Bus Selector/7 -> Logical Operator/1  "<IO191_DI_CH9_Bremspedal_1>"
  Bus Selector/8 -> Logical Operator1/1  "<IO191_DI_CH10_Bremspedal_2>"
  Logical Operator/1 -> AND2/6
  Logical Operator1/1 -> AND2/7
  Unit Delay/1 -> Logical Operator/2, Logical Operator1/2
  EMV Filter/1(Out) -> 1s Tastersperre/1(In)

== system D_20210914_Modell_Inbetriebnahme_BreakOutBox_Jetson/Freigabe/Totmann ==
  Bus_In : Inport
  AND : Logic  AllPortsSameDT=off  OutDataTypeStr=boolean
  Bus Selector : BusSelector  OutputSignals=IO191_Out.IO191_DI.IO191_DI_CH12_Totmann_Taster_1,IO191_Out.IO191_DI.IO191_DI_CH13_Totmann_Taster_2
  Compare To Constant : simulink/Logic and Bit Operations/Compare To Constant  relop===  const=1  OutDataTypeStr=boolean
  Compare To Constant1 : simulink/Logic and Bit Operations/Compare To Constant  relop===  const=0  OutDataTypeStr=boolean
  Compare To Constant2 : simulink/Logic and Bit Operations/Compare To Constant  relop=<  const=30  OutDataTypeStr=boolean
  Compare To Constant3 : simulink/Logic and Bit Operations/Compare To Constant  relop=<=  const=45  OutDataTypeStr=boolean
  Constant : Constant
  Constant1 : Constant  Value=0
  Constant2 : Constant
  Integrator : Integrator  ExternalReset=rising
  Pulse Generator : DiscretePulseGenerator  PulseType=Time based  PulseWidth=75
  Switch : Switch  Criteria=u2 > Threshold
  Switch1 : Switch  Criteria=u2 > Threshold
  Switch2 : Switch  Criteria=u2 > Threshold
  Totmann_Freigabe : Outport
  Totmann_LED : Outport  Port=2
  wires:
  Bus_In/1 -> Bus Selector/1
  Bus Selector/1 -> Compare To Constant/1  "<IO191_DI_CH12_Totmann_Taster_1>"
  Bus Selector/2 -> Compare To Constant1/1  "<IO191_DI_CH13_Totmann_Taster_2>"
  Compare To Constant/1 -> AND/1
  Compare To Constant1/1 -> AND/2
  Constant/1 -> Switch/1, Integrator/1
  AND/1 -> Integrator/2
  Switch/1 -> Switch1/1
  Integrator/1 -> Compare To Constant3/1, Compare To Constant2/1
  Compare To Constant2/1 -> Switch/2
  Pulse Generator/1 -> Switch/3
  Switch1/1 -> Totmann_LED/1
  Compare To Constant3/1 -> Switch2/2, Switch1/2
  Constant1/1 -> Switch2/3, Switch1/3
  Switch2/1 -> Totmann_Freigabe/1
  Constant2/1 -> Switch2/1

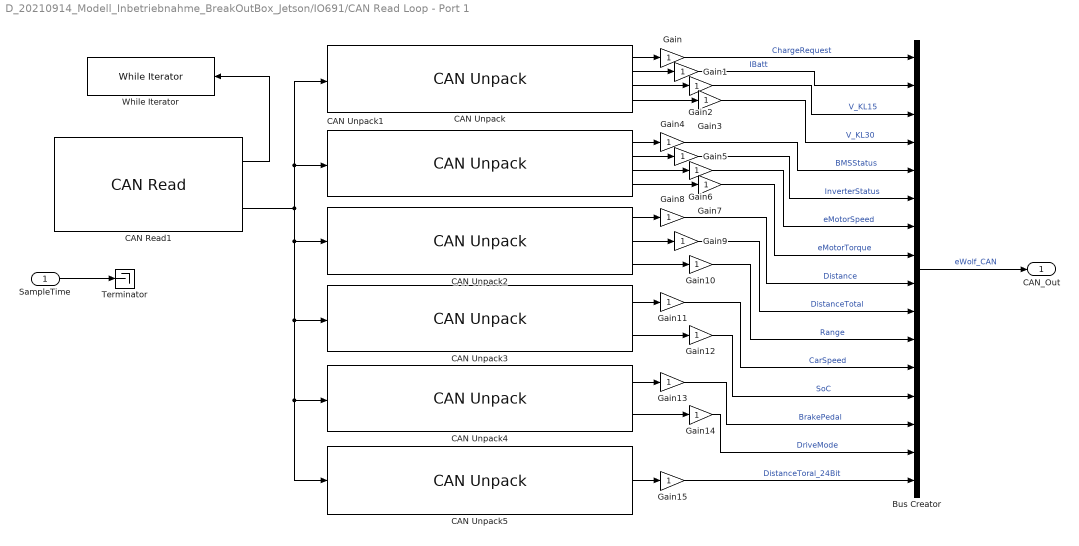
== system D_20210914_Modell_Inbetriebnahme_BreakOutBox_Jetson/IO691/CAN Read Loop - Port 1 ==
  SampleTime : Inport
  Bus Creator : BusCreator  Inputs=16
  CAN Read1 : speedgoatlib_IO691/CAN Read  id=1  ts=-1  channel=2  messageType=CAN  canType=CAN (HS)  BusOutput=off  initValues=[691 1 -1 1 1 1 0]
      settings: SourceProductName=Simulink Real-Time: Speedgoat Library
  CAN Unpack : canmsglib/CAN Unpack  CANdbFile=Delta2_MeasurementCAN.dbc  MsgList=VCU2DL2  MsgName=VCU2DL2  MsgIDType=Standard (11-bit identifier)  MsgIdentifier=1041  MsgLength=8  SignalInfo={'ChargeRequest','56','16','BE','unsigned','Standard','0','0.01','0','0','655.35';'IBatt','8','16','BE','signed','Standard','0','0.01','0','-32767','32768';'V_KL15','40','16','BE','unsigned','Standard','0','0.01','0','0','65535';'V_KL30','24','16','BE','unsigned','Standard','0','0.01','0','0','65535'}  IDPort=off  TimestampPort=off  ErrorPort=off  RemotePort=off  LengthPort=off  StatusPort=off  ApplyMinMax=off
      settings: SourceProductBaseCode=ME,XP,VN  DataFormat=CANdb specified signals
  CAN Unpack1 : canmsglib/CAN Unpack  CANdbFile=Delta2_MeasurementCAN.dbc  MsgList=VCU2DL3  MsgName=VCU2DL3  MsgIDType=Standard (11-bit identifier)  MsgIdentifier=1045  MsgLength=8  SignalInfo={'BMSStatus','56','16','BE','unsigned','Standard','0','1','0','0','65535';'InverterStatus','40','16','BE','unsigned','Standard','0','1','0','0','65535';'eMotorSpeed','24','16','BE','signed','Standard','0','0.01','0','-32767','32768';'eMotorTorque','8','16','BE','signed','Standard','0','0.01','0','-32767','32768'}  IDPort=off  TimestampPort=off  ErrorPort=off  RemotePort=off  LengthPort=off  StatusPort=off  ApplyMinMax=off
      settings: SourceProductBaseCode=ME,XP,VN  DataFormat=CANdb specified signals
  CAN Unpack2 : canmsglib/CAN Unpack  CANdbFile=Delta2_MeasurementCAN.dbc  MsgList=VCU2DL4  MsgName=VCU2DL4  MsgIDType=Standard (11-bit identifier)  MsgIdentifier=1056  MsgLength=8  SignalInfo={'Distance','24','16','BE','unsigned','Standard','0','0.1','0','0','65535';'DistanceTotal','56','32','BE','unsigned','Standard','0','0.1','0','0','429496729.5';'Range','8','16','BE','unsigned','Standard','0','0.1','0','0','65535'}  IDPort=off  TimestampPort=off  ErrorPort=off  RemotePort=off  LengthPort=off  StatusPort=off  ApplyMinMax=off
      settings: SourceProductBaseCode=ME,XP,VN  DataFormat=CANdb specified signals
  CAN Unpack3 : canmsglib/CAN Unpack  CANdbFile=Delta2_MeasurementCAN.dbc  MsgList=VCU2DL5  MsgName=VCU2DL5  MsgIDType=Standard (11-bit identifier)  MsgIdentifier=1057  MsgLength=8  SignalInfo={'CarSpeed','16','16','BE','unsigned','Standard','0','0.1','0','0','65535';'SoC','0','8','BE','unsigned','Standard','0','0.5','0','0','255'}  IDPort=off  TimestampPort=off  ErrorPort=off  RemotePort=off  LengthPort=off  StatusPort=off  ApplyMinMax=off
      settings: SourceProductBaseCode=ME,XP,VN  DataFormat=CANdb specified signals
  CAN Unpack4 : canmsglib/CAN Unpack  CANdbFile=Delta2_MeasurementCAN.dbc  MsgList=VCU2DL7  MsgName=VCU2DL7  MsgIDType=Standard (11-bit identifier)  MsgIdentifier=1059  MsgLength=8  SignalInfo={'BrakePedal','8','1','BE','unsigned','Standard','0','1','0','0','1';'DriveMode','0','8','BE','unsigned','Standard','0','1','0','0','255'}  IDPort=off  TimestampPort=off  ErrorPort=off  RemotePort=off  LengthPort=off  StatusPort=off  ApplyMinMax=off
      settings: SourceProductBaseCode=ME,XP,VN  DataFormat=CANdb specified signals
  CAN Unpack5 : canmsglib/CAN Unpack  CANdbFile=Delta2_MeasurementCAN.dbc  MsgList=VCU_0x400  MsgName=VCU_0x400  MsgIDType=Standard (11-bit identifier)  MsgIdentifier=1024  MsgLength=8  SignalInfo={'DistanceTotal_24Bit','56','24','BE','unsigned','Standard','0','1','0','0','16777215'}  IDPort=off  TimestampPort=off  ErrorPort=off  RemotePort=off  LengthPort=off  StatusPort=off  ApplyMinMax=off
      settings: SourceProductBaseCode=ME,XP,VN  DataFormat=CANdb specified signals
  Gain{,1..15} (16 alike) : Gain
  Terminator : Terminator
  While Iterator : WhileIterator  MaxIters=501  WhileBlockType=do-while
  CAN_Out : Outport
  wires:
  SampleTime/1 -> Terminator/1
  CAN Read1/1 -> While Iterator/1
  CAN Read1/2 -> CAN Unpack5/1, CAN Unpack4/1, CAN Unpack3/1, CAN Unpack2/1, CAN Unpack1/1, CAN Unpack/1
  CAN Unpack/1 -> Gain/1
  CAN Unpack/2 -> Gain1/1
  CAN Unpack/3 -> Gain2/1
  CAN Unpack/4 -> Gain3/1
  CAN Unpack1/1 -> Gain4/1
  CAN Unpack1/2 -> Gain5/1
  CAN Unpack1/3 -> Gain6/1
  CAN Unpack1/4 -> Gain7/1
  CAN Unpack2/1 -> Gain8/1
  CAN Unpack2/2 -> Gain9/1
  CAN Unpack2/3 -> Gain10/1
  CAN Unpack3/1 -> Gain11/1
  CAN Unpack3/2 -> Gain12/1
  CAN Unpack4/1 -> Gain13/1
  CAN Unpack4/2 -> Gain14/1
  CAN Unpack5/1 -> Gain15/1
  Gain/1 -> Bus Creator/1  "ChargeRequest"
  Gain1/1 -> Bus Creator/2  "IBatt"
  Gain2/1 -> Bus Creator/3  "V_KL15"
  Gain3/1 -> Bus Creator/4  "V_KL30"
  Gain4/1 -> Bus Creator/5  "BMSStatus"
  Gain5/1 -> Bus Creator/6  "InverterStatus"
  Gain6/1 -> Bus Creator/7  "eMotorSpeed"
  Gain7/1 -> Bus Creator/8  "eMotorTorque"
  Gain8/1 -> Bus Creator/9  "Distance"
  Gain9/1 -> Bus Creator/10  "DistanceTotal"
  Gain10/1 -> Bus Creator/11  "Range"
  Gain11/1 -> Bus Creator/12  "CarSpeed"
  Gain12/1 -> Bus Creator/13  "SoC"
  Gain13/1 -> Bus Creator/14  "BrakePedal"
  Gain14/1 -> Bus Creator/15  "DriveMode"
  Gain15/1 -> Bus Creator/16  "DistanceToral_24Bit"
  Bus Creator/1 -> CAN_Out/1  "eWolf_CAN"
